simulink model "SMA_valve"  (R2018a)
settings: Solver=VariableStepAuto  StartTime=0.0  StopTime=10.0  RelTol=1e-3
undefined symbols (not defined in the file or in its folder): param_factor
settings Model: Creator=tim  LastModifiedBy=tim

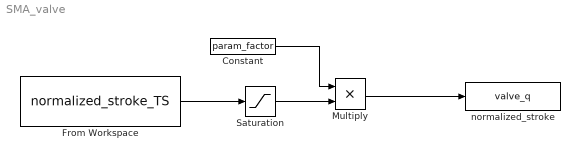
== system SMA_valve ==
  Constant : Constant  Value=param_factor
  From Workspace : FromWorkspace  VariableName=normalized_stroke_TS  SampleTime=0
  Multiply : Product
  Saturation : Saturate  UpperLimit=1  LowerLimit=0
  normalized_stroke : ToWorkspace  VariableName=valve_q  SampleTime=-1
  wires:
  From Workspace/1 -> Saturation/1
  Saturation/1 -> Multiply/2
  Constant/1 -> Multiply/1
  Multiply/1 -> normalized_stroke/1
